simulink model "compensadorFeedforward"  (R2022a)
settings: Solver=VariableStepAuto  StartTime=0.0  StopTime=10.0  RelTol=1e-3
values from neighbouring files (symbols this model uses):
  Beff = 1    [scriptLista3.m]
  Jeff = 0.15    [scriptLista3.m]
  K = 1    [scriptLista3.m]
  Kp = Jeff*(omega_n^2)/K    (= 3.75)    [scriptLista3.m]
settings Model: Creator=vfton  LastModifiedBy=vfton

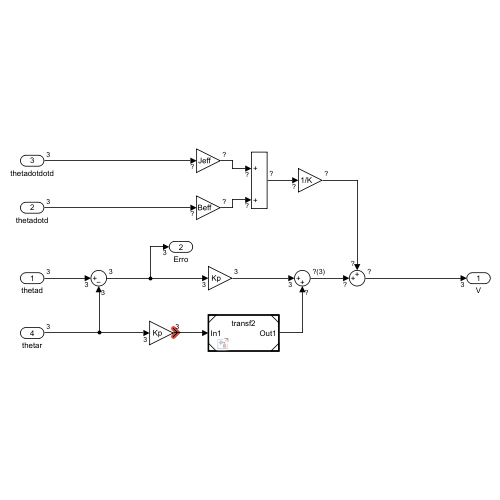
[thumbnail: Simulink's stored preview of the top-level diagram]
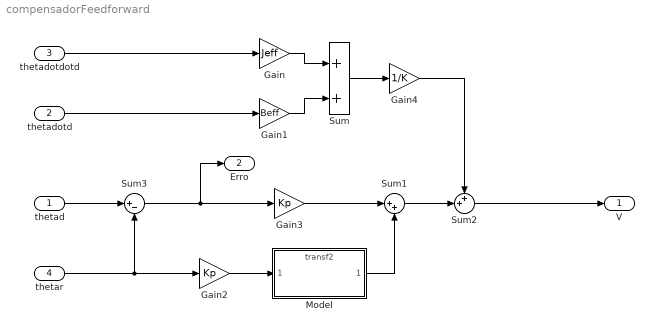
== system compensadorFeedforward ==
  thetad : Inport  PortDimensions=3
  thetadotd : Inport  Port=2  PortDimensions=3
  thetadotdotd : Inport  Port=3  PortDimensions=3
  thetar : Inport  Port=4  PortDimensions=3
  Gain : Gain  Gain=Jeff
  Gain1 : Gain  Gain=Beff
  Gain2 : Gain  Gain=Kp
  Gain3 : Gain  Gain=Kp
  Gain4 : Gain  Gain=1/K
  Model : ModelReference  ModelNameDialog=transf2.slx  SimulationMode=Normal  ModelReferenceVersion=1.2
  Sum : Sum  Inputs=|+|||+
  Sum1 : Sum  Inputs=|++
  Sum2 : Sum  Inputs=++|
  Sum3 : Sum  Inputs=|+-
  V : Outport  PortDimensions=3
  Erro : Outport  Port=2  PortDimensions=3
  wires:
  Gain/1 -> Sum/1
  Gain1/1 -> Sum/2
  Sum1/1 -> Sum2/2
  Sum/1 -> Gain4/1
  Model/1 -> Sum1/2
  Gain2/1 -> Model/1
  Gain3/1 -> Sum1/1
  thetadotdotd/1 -> Gain/1
  thetadotd/1 -> Gain1/1
  thetar/1 -> Sum3/2, Gain2/1
  thetad/1 -> Sum3/1
  Sum3/1 -> Erro/1, Gain3/1
  Sum2/1 -> V/1
  Gain4/1 -> Sum2/1
